simulink subsystem "LecturaEncoders"  (R2021b)
settings: Solver=VariableStepAuto  StartTime=0.0  StopTime=10.0  RelTol=1e-3
libraries: simulink x1
settings Model: Creator=ferna  LastModifiedBy=Mauri

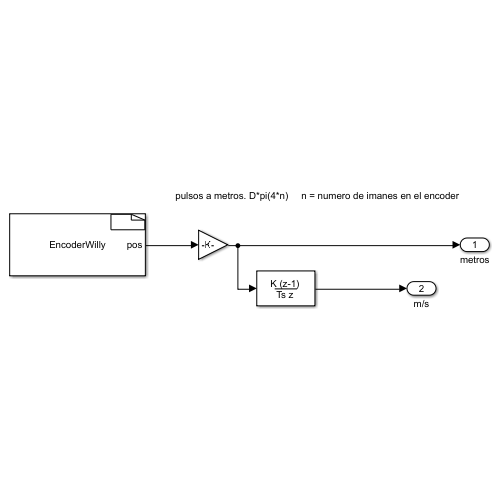
[thumbnail: Simulink's stored preview of the top-level diagram]
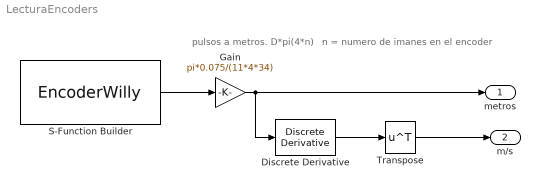
== system LecturaEncoders ==
  note: pulsos a metros. D*pi(4*n)
  note: n = numero de imanes en el encoder
  Discrete Derivative : simulink/Discrete/Discrete Derivative  gainval=1.0  ICPrevScaledInput=0.0  OutMin=[]  OutMax=[]  OutDataType=fixdt(1, 16)  OutScaling=2^-10  DoSatur=off
  Gain : Gain  Gain=pi*0.075/(11*4*34)  ParamDataTypeStr=double
  S-Function Builder : S-Function  FunctionName=EncoderWilly  Parameters=uint8(2),uint8(3),18,19  SFunctionModules=EncoderWilly_wrapper  SFunctionDeploymentMode=off  EnableBusSupport=off  mask(S-Function Builder){}
      mask help: Simulink:masks:SFunctionBuilder_MD
      mask init:
      | val = [[.9  0.75 0.75 1 1 .9 .9 1]',[1 1 0.75 0.75 .9 .9 1 .9]'];try , sys = get_param(gcb,'SfunBuilderFcnName');if isempty(sys), sys = get_param(gcb,'FunctionName'); end,catch, sys = get_param(gcb,'FunctionName'); end
      settings: CopyFcn=set_param(gcbh,'LinkStatus','none')  OpenFcn=sfunctionwizard(gcbh)
      mask Display: plot(val(:,1),val(:,2)),disp(sys),port_label('output',1,'pos')
  Transpose : Math  Operator=transpose  SaturateOnIntegerOverflow=on
  metros : Outport
  m/s : Outport  Port=2
  wires:
  Discrete Derivative/1 -> Transpose/1
  Gain/1 -> Discrete Derivative/1, metros/1
  S-Function Builder/1 -> Gain/1
  Transpose/1 -> m/s/1
